simulink model "Ratchet"  (R2022a)
settings: Solver=ode45  StartTime=0.0  StopTime=10.0  MaxStep=0.01  RelTol=1e-3
libraries: fl_lib x8, nesl_utility x4, sdl_lib x2
settings Model: Creator=Mohammad Almalak  LastModifiedBy=Mohammad Almalak

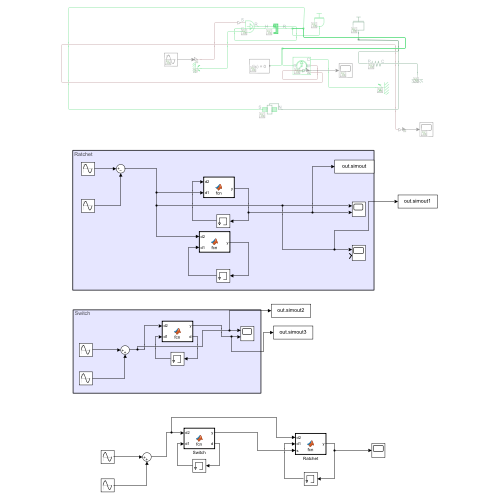
[thumbnail: Simulink's stored preview of the top-level diagram]
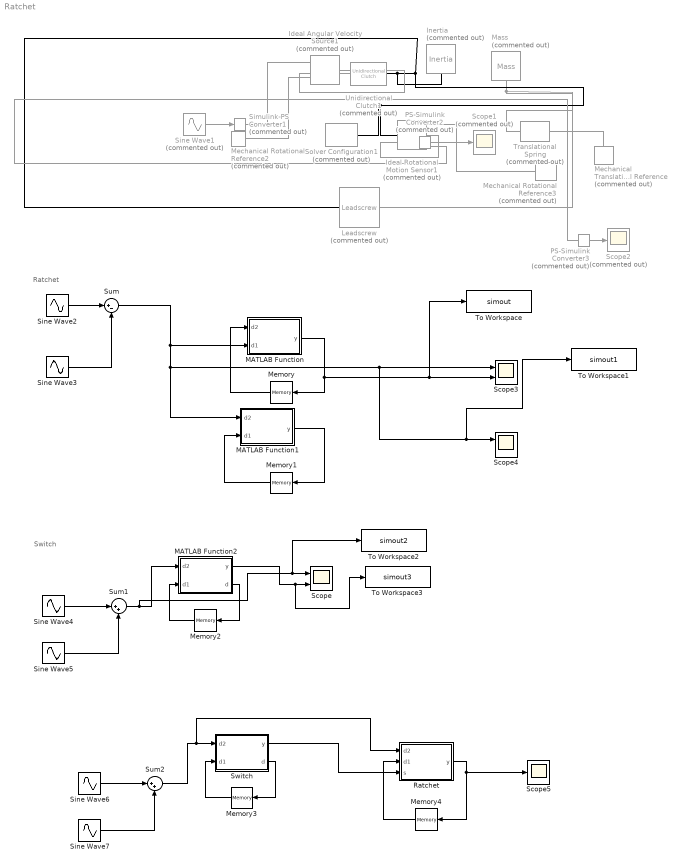
== system Ratchet ==
  note: Switch
  note: Ratchet
  Ideal Angular Velocity Source1 : fl_lib/Mechanical/Mechanical Sources/Ideal Angular Velocity Source  Commented=on
      settings: SourceProductBaseCode=PW,SS,VE
  Ideal Rotational Motion Sensor1 : fl_lib/Mechanical/Mechanical Sensors/Ideal Rotational Motion Sensor  Commented=on  wrap_angle=simscape.enum.onoff.off  offset=0 rad
      settings: SourceProductBaseCode=PW,SS,VE
  Inertia : fl_lib/Mechanical/Rotational Elements/Inertia  Commented=on  inertia=0.01 kg*m^2  num_ports=foundation.enum.numPorts2.one  w_specify=off  w_priority=High  w=0 rad/s  w_nominal_specify=off  w_nominal_unit=rad/s  w_nominal_value=1  t_specify=off  t_priority=None  t=0 N*m  t_nominal_specify=off  t_nominal_unit=N*m  t_nominal_value=1
      settings: SourceProductBaseCode=PW,SS,VE
  Leadscrew : sdl_lib/Gears/Rotational- Translational/Leadscrew  Commented=on  Lead=0.015 m  helix_type=sdl.enum.handedness.right  friction_model=sdl.enum.gear_friction.none  friction_parameterization=sdl.enum.frictionParameterization.geometry  lambda=15 deg  alpha=14.5 deg  fr_coeff=0.08  eff_sn=0.75  eff_ns=0.45  temperature_TLU=[280, 300, 320] K  efficiency_sn_TLU=[.75, .65, .6]  efficiency_ns_TLU=[.5, .45, .4]  pwr_thr=0.001 W  mu_visc=0 N*m*s/rad  thermal_mass=50 J/K  temperature_specify=off  temperature_priority=High  temperature=300 K  temperature_nominal_specify=off  temperature_nominal_unit=K  temperature_nominal_value=1
      settings: SourceProductBaseCode=LD  InternalSimscapePortConfiguration="{\"Bottom\":[],\"Left\":[{\"id\":\"S\",\"label\":\"S\",\"type\":\"foundation.mechanical.rotational.rotational\"}],\"Right\":[{\"id\":\"N\",\"label\":\"N\",\"type\":\"foundation.mechanical.translational.translational\"}],\"Top\":[]}"
  MATLAB Function : MATLAB Function  TreatAsAtomicUnit=on
  MATLAB Function1 : MATLAB Function  TreatAsAtomicUnit=on
  MATLAB Function2 : MATLAB Function  TreatAsAtomicUnit=on
  Mass : fl_lib/Mechanical/Translational Elements/Mass  Commented=on  mass=1 kg  num_ports=foundation.enum.numPorts2.one  v_specify=off  v_priority=High  v=0 m/s  v_nominal_specify=off  v_nominal_unit=m/s  v_nominal_value=1  f_specify=off  f_priority=None  f=0 N  f_nominal_specify=off  f_nominal_unit=N  f_nominal_value=1
      settings: SourceProductBaseCode=PW,SS,VE
  Mechanical Rotational Reference2 : fl_lib/Mechanical/Rotational Elements/Mechanical Rotational Reference  Commented=on
      settings: SourceProductBaseCode=PW,SS,VE
  Mechanical Rotational Reference3 : fl_lib/Mechanical/Rotational Elements/Mechanical Rotational Reference  Commented=on
      settings: SourceProductBaseCode=PW,SS,VE
  Mechanical Translational Reference : fl_lib/Mechanical/Translational Elements/Mechanical Translational Reference  Commented=on
      settings: SourceProductBaseCode=PW,SS,VE
  Memory{,1..4} (5 alike) : Memory
  PS-Simulink Converter2 : nesl_utility/PS-Simulink Converter  Commented=on  PhysicalDomain=network_engine_domain  SubClassName=ps_output  LeftPortType=input  RightPortType=output  PseudoPeriodic=off  Frequencies=[]  VectorFormat=inherit  Unit=inherit  AffineConversion=off
      settings: SourceProductBaseCode=SS,PW,VE
  PS-Simulink Converter3 : nesl_utility/PS-Simulink Converter  Commented=on  PhysicalDomain=network_engine_domain  SubClassName=ps_output  LeftPortType=input  RightPortType=output  PseudoPeriodic=off  Frequencies=[]  VectorFormat=inherit  Unit=inherit  AffineConversion=off
      settings: SourceProductBaseCode=SS,PW,VE
  Ratchet : MATLAB Function  TreatAsAtomicUnit=on
  Scope : Scope  NumInputPorts=2
  Scope1 : Scope  Commented=on
  Scope2 : Scope  Commented=on
  Scope3 : Scope  NumInputPorts=2
  Scope4 : Scope  NumInputPorts=2
  Scope5 : Scope
  Simulink-PS Converter1 : nesl_utility/Simulink-PS Converter  Commented=on  PhysicalDomain=network_engine_domain  SubClassName=ps_input  LeftPortType=input  RightPortType=output  PseudoPeriodic=off  Frequencies=[]  NoiseDistribution=none  NoiseParameters=[]  Unit=rad/s  AffineConversion=off  FilteringAndDerivatives=provide  SimscapeFilterOrder=1  InputFilterTimeConstant=0.001  UdotUserProvided=0
      settings: SourceProductBaseCode=SS,PW,VE
  Sine Wave1 : Sin  Commented=on  SampleTime=0
  Sine Wave2 : Sin  Frequency=0.33  SampleTime=0
  Sine Wave3 : Sin  Amplitude=2  Frequency=3  SampleTime=0
  Sine Wave4 : Sin  Frequency=0.33  SampleTime=0
  Sine Wave5 : Sin  Amplitude=2  Frequency=3  SampleTime=0
  Sine Wave6 : Sin  Frequency=0.33  SampleTime=0
  Sine Wave7 : Sin  Amplitude=2  Frequency=3  SampleTime=0
  Solver Configuration1 : nesl_utility/Solver Configuration  Commented=on  PhysicalDomain=network_engine_domain  SubClassName=solver  LeftPortType=input  RightPortType=generic  Tones=[]  Harmonics=[]  SimulateNoise=off  Profile=off  UseLocalSampling=off  EnableSwitchedLinearOptims=on  FrequencyDomain=off  UseCCode=off  RelTol=0.001  AbsTol=0.001  MinStep=1e-09  ToWorkspace=off  RevertToSquareIcSolve=off  NumHomotopyIterations=100  PhasorMode=off  PhasorModeNumHarmonics=1  IndexReductionMethod=DerivativeReplacement  DoDC=off  ResidualTolerance=1e-09  UseLocalSolver=off  LocalSolverChoice=NE_BACKWARD_EULER_ADVANCER  LocalSolverSampleTime=0.001  DoFixedCost=off  MaxNonlinIter=3  MaxModeIter=2  ComputeImpulses=off  ImpulseIterations=2  LinearAlgebra=auto  LinearAlgebraNumThread=0  EquationFormulation=NE_TIME_EF  DelaysMemoryBudget=1024  AutomaticFiltering=on  FilteringTimeConstant=0.001  PartitionStorageMethod=AS_NEEDED  PartitionMemoryBudget=1024  PartitionMethod=ROBUST
      settings: SourceProductBaseCode=SS,PW,VE
  Sum : Sum  Inputs=|+-
  Sum1 : Sum  Inputs=|++
  Sum2 : Sum  Inputs=|++
  Switch : MATLAB Function  TreatAsAtomicUnit=on
  To Workspace : ToWorkspace  VariableName=simout  SaveFormat=Timeseries  SampleTime=-1
  To Workspace1 : ToWorkspace  VariableName=simout1  SaveFormat=Timeseries  SampleTime=-1
  To Workspace2 : ToWorkspace  VariableName=simout2  SaveFormat=Timeseries  SampleTime=-1
  To Workspace3 : ToWorkspace  VariableName=simout3  SaveFormat=Timeseries  SampleTime=-1
  Translational Spring : fl_lib/Mechanical/Translational Elements/Translational Spring  Commented=on  spr_rate=1000 N/m  v_specify=off  v_priority=None  v=0 m/s  v_nominal_specify=off  v_nominal_unit=m/s  v_nominal_value=1  f_specify=off  f_priority=None  f=0 N  f_nominal_specify=off  f_nominal_unit=N  f_nominal_value=1  x_specify=off  x_priority=High  x=0 m  x_nominal_specify=off  x_nominal_unit=m  x_nominal_value=1
      settings: SourceProductBaseCode=PW,SS,VE
  Unidirectional Clutch1 : sdl_lib/Clutches/Unidirectional Clutch  Commented=on  transmission_direction=sdl.enum.hubRingDirection.positive  initial_state_locked=sdl.enum.initial_lock.unlocked
      settings: SourceProductBaseCode=LD  InternalSimscapePortConfiguration="{\"Bottom\":[],\"Left\":[{\"id\":\"H\",\"label\":\"H\",\"type\":\"foundation.mechanical.rotational.rotational\"}],\"Right\":[{\"id\":\"R\",\"label\":\"R\",\"type\":\"foundation.mechanical.rotational.rotational\"}],\"Top\":[]}"
  wires:
  PS-Simulink Converter2/1 -> Scope1/1
  Sine Wave1/1 -> Simulink-PS Converter1/1
  PS-Simulink Converter3/1 -> Scope2/1
  Sine Wave2/1 -> Sum/1
  Memory1/1 -> MATLAB Function1/2(d1)
  Sum/1 -> MATLAB Function/2(d1), To Workspace1/1, Scope4/1, Scope3/1, MATLAB Function1/1(d2)
  Sine Wave3/1 -> Sum/2
  MATLAB Function1/1(y) -> Memory1/1
  Memory/1 -> MATLAB Function/1(d2)
  MATLAB Function/1(y) -> To Workspace/1, Scope3/2, Memory/1
  Sine Wave5/1 -> Sum1/2
  MATLAB Function2/2(d) -> Memory2/1
  MATLAB Function2/1(y) -> To Workspace3/1, Scope/2
  Sum1/1 -> To Workspace2/1, Scope/1, MATLAB Function2/1(d2)
  Sine Wave4/1 -> Sum1/1
  Memory2/1 -> MATLAB Function2/2(d1)
  Memory3/1 -> Switch/2(d1)
  Sine Wave7/1 -> Sum2/2
  Switch/2(d) -> Memory3/1
  Sine Wave6/1 -> Sum2/1
  Sum2/1 -> Ratchet/1(d2), Switch/1(d2)
  Switch/1(y) -> Ratchet/3(s)
  Memory4/1 -> Ratchet/2(d1)
  Ratchet/1(y) -> Scope5/1, Memory4/1
  connections:
  Mass/LConn1 -- Leadscrew/RConn1 -- Translational Spring/LConn1
  Unidirectional Clutch1/RConn1 -- Solver Configuration1/RConn1 -- Ideal Rotational Motion Sensor1/LConn1 -- Leadscrew/LConn1 -- Inertia/LConn1
  Mechanical Translational Reference/LConn1 -- Translational Spring/RConn1
  Ideal Rotational Motion Sensor1/RConn3 -- PS-Simulink Converter3/LConn1
  Simulink-PS Converter1/RConn1 -- Ideal Angular Velocity Source1/RConn1
  Ideal Angular Velocity Source1/LConn1 -- Unidirectional Clutch1/LConn1
  Mechanical Rotational Reference2/LConn1 -- Ideal Angular Velocity Source1/RConn2
  PS-Simulink Converter2/LConn1 -- Ideal Rotational Motion Sensor1/RConn2
  Mechanical Rotational Reference3/LConn1 -- Ideal Rotational Motion Sensor1/RConn1

== matlab function Ratchet/MATLAB Function ==
  data: d2 input; d1 input; y output
function y = fcn(d2,d1)

if d2>d1
    y=d2;
else
    y=d1;
end

== matlab function Ratchet/MATLAB Function2 ==
  data: d2 input; d1 input; y output; d output
function [y,d] = fcn(d2,d1)

if d2>d1
    y=1;
else
    y=0;
end
d=d2;

== matlab function Ratchet/Ratchet ==
  data: d2 input; d1 input; y output; s input
function y = fcn(d2,d1,s)
if s==1
    if d2>d1
    y=d2;
        else
    y=d1;
    end
else 

    if d1>d2
        y=d2;
    else
        y=d1;
    end


end

== matlab function Ratchet/Switch ==
  data: d2 input; d1 input; y output; d output
function [y,d] = fcn(d2,d1)

if d2>d1
    y=1;
else
    y=0;
end
d=d2;

== matlab function Ratchet/MATLAB Function1 ==
  data: d2 input; d1 input; y output
function y = fcn(d2,d1)

if d1>d2
    y=d2;
else
    y=d1;
end
